simulink model "motor_controlsys1"  (R2023a)
settings: Solver=VariableStepAuto  StartTime=0.0  StopTime=400  RelTol=1e-3
libraries: simulink x1
settings Model: Creator=User  LastModifiedBy=User

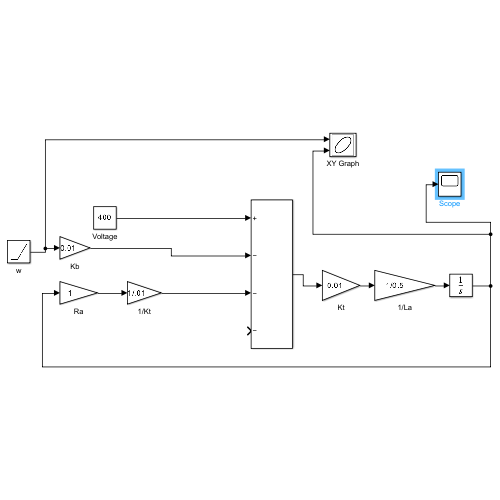
[thumbnail: Simulink's stored preview of the top-level diagram]
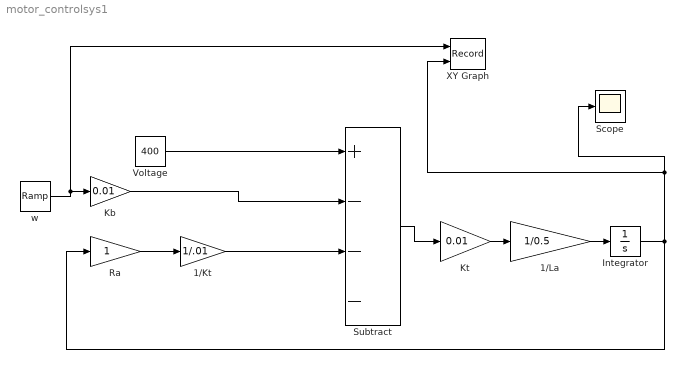
== system motor_controlsys1 ==
  1/Kt : Gain  Gain=1/.01
  1/La : Gain  Gain=1/0.5
  Integrator : Integrator
  Kb : Gain  Gain=0.01
  Kt : Gain  Gain=0.01
  Ra : Gain
  Scope : Scope
  Subtract : Sum  Inputs=+---
  Voltage : Constant  Value=400
  XY Graph : Record  FileSettingsInternal="{\"entries\":[{\"content\":{\"excelSettings\":{\"content\":{},\"type\":\"Streamout.ExcelSettings\"}},\"type\":\"Streamout.FileSettingStorage\",\"uuid\":\"f1e0ee9e-a43b-481a-80f7-9086f16c0496\"}],\"packageUris\":[\"http://schema.mathworks.com/mf0/streamout_blocks/R2020a\"],\"version\":\"1.0\"}"  Layout=[1 1]  SignalsInternal="{\"entries\":[{\"content\":{\"signals\":[{\"content\":{\"blockPath\":[\"motor_controlsys1/XY Graph\"],\"dimensions\":[1],\"domain\":\"motor_controlsys1/XY Graph\",\"lineColor\":\"#a2142f\",\"plots\":[1],\"port\":1,\"sid\":[\"\"],\"signalID\":75,\"signalName\":\"w\"},\"type\":\"RecordBlkView.Signal\",\"uuid\":\"14a83f1c-c5ba-4110-b0e2-ea2992762497\"},{\"content\":{\"blockPath\":[\"motor_controlsys1/XY Graph\"],\"dimensions\":[1],\"domain\":\"motor_controlsys1/XY Graph\",\"lineColor\":\"#139fff\",\"plots\":[1],\"port\":2,\"sid\":[\"\"],\"signalID\":79,\"signalName\":\"Integrator\"},\"type\":\"RecordBlkView.Signal\",\"uuid\":\"8da38879-d327-4a6c-af20-a8e003e66a7a\"}]},\"type\":\"RecordBlkView.InputSignals\",\"uuid\":\"f58a3f07-b9ef-4d61-9b36-2d40eead3b33\"}],\"packageUris\":[\"http://schema.mathworks.com/mf0/streamout_blocks/R2020a\"],\"version\":\"1.0\"}"  VisualizationBindings="{\"xyplotplugin\":{\"info\":[{\"series\":[{\"bindingParametersList\":[{\"parameter\":\"X-Axis\",\"signalID\":75,\"signalName\":\"w\"},{\"parameter\":\"Y-Axis\",\"signalID\":79,\"signalName\":\"Integrator\"}],\"seriesID\":9085}],\"subplotID\":1}]}}"  CompatibilityTag=XY
  w : simulink/Sources/Ramp  slope=5  start=0  InitialOutput=0
  wires:
  Voltage/1 -> Subtract/1
  1/Kt/1 -> Subtract/3
  Ra/1 -> 1/Kt/1
  1/La/1 -> Integrator/1
  Integrator/1 -> Ra/1, XY Graph/2, Scope/1
  Subtract/1 -> Kt/1
  Kt/1 -> 1/La/1
  Kb/1 -> Subtract/2
  w/1 -> XY Graph/1, Kb/1
